simulink model "second_equation_model_fixed"  (R2024a)
settings: Solver=VariableStepAuto  StartTime=0.0  StopTime=10.0  RelTol=1e-3
settings Model: Creator=andrey  LastModifiedBy=andrey

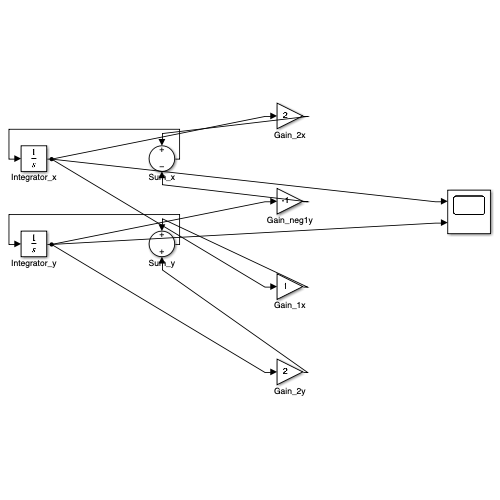
[thumbnail: Simulink's stored preview of the top-level diagram]
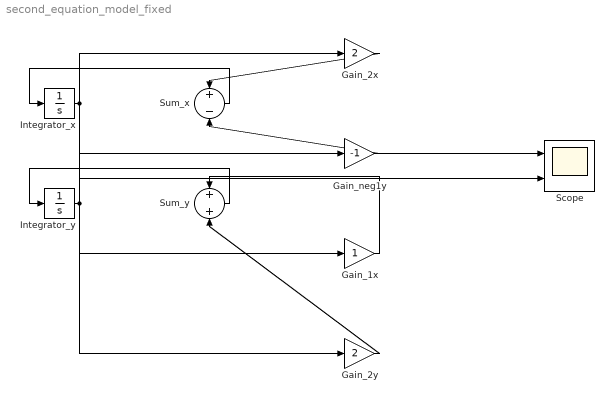
== system second_equation_model_fixed ==
  Gain_1x : Gain
  Gain_2x : Gain  Gain=2
  Gain_2y : Gain  Gain=2
  Gain_neg1y : Gain  Gain=-1
  Integrator_x : Integrator  InitialCondition=-1
  Integrator_y : Integrator
  Scope : Scope  NumInputPorts=2
  Sum_x : Sum  Inputs=+-
  Sum_y : Sum
  wires:
  Integrator_x/1 -> Gain_2x/1, Gain_1x/1, Scope/1
  Integrator_y/1 -> Gain_neg1y/1, Gain_2y/1, Scope/2
  Gain_2x/1 -> Sum_x/1
  Gain_neg1y/1 -> Sum_x/2
  Sum_x/1 -> Integrator_x/1
  Gain_1x/1 -> Sum_y/1
  Gain_2y/1 -> Sum_y/2
  Sum_y/1 -> Integrator_y/1
